simulink model "syncMachVsSwing_sim"  (R2014b)
settings: Solver=ode45  SolverMode=SingleTasking  StartTime=0.0  StopTime=10  MaxStep=0.001  RelTol=0.0001
values from neighbouring files (symbols this model uses):
  cc1 = 2*Ld*Lff - 3*Laf^2    (= 0.0506605918212)    [syncMachVsSwing.m]
  Ert = mpcA.gen([2 3],VG)*baseV    [ex14busSGandPV.m]    (also in ex7busLongLine.m = 24200; exDroopA.m = mpc.bus(ssgen,VM).*baseV(ssgen); exDroopB.m = mpc.bus(ssgen,VM).*baseV(ssgen); exSyncGenPVinv.m = Ert( [1:(synrp-1),(synrp+1):end]  ))
  If_dc = 0.2*Prt./Ert    [ex14busSGandPV.m]    (also in ex7busLongLine.m = Prt./(60*Vf_dc); exDroopA.m = Prt./(60*Vf_dc); exDroopB.m = Prt./(60*Vf_dc); exSyncGenPVinv.m)
  Kd = KD_GAIN_CNST*J*ws    [ex14busSGandPV.m]    (also in ex2busStability.m = 24000; ex7busLongLine.m; ex9busSG.m; exDroopA.m)
  L0 = 0.1*Ld    [ex14busSGandPV.m]    (also in ex7busLongLine.m; exDroopA.m; exDroopB.m; exSyncGenPVinv.m)
  Laf = (2^0.5)*Ert./(ws*If_dc)    [ex14busSGandPV.m]    (also in ex7busLongLine.m; exDroopA.m; exDroopB.m; exSyncGenPVinv.m = (2^0.5)*5*Ert.^2./(ws*Prt))
  Ld = 0.6*Lpu    [ex14busSGandPV.m]    (also in ex7busLongLine.m = 0.3*Lpu; exDroopA.m = 0.3*Lpu; exDroopB.m = 0.3*Lpu; exSyncGenPVinv.m)
  Lff = 2*Laf.^2./Ld    [ex14busSGandPV.m]    (also in ex7busLongLine.m; exDroopA.m; exDroopB.m; exSyncGenPVinv.m)
  Lq = Ld    [ex14busSGandPV.m]    (also in ex7busLongLine.m; exDroopA.m; exDroopB.m; exSyncGenPVinv.m)
  Ls = (Ld+Lq)/2    [ex14busSGandPV.m]    (also in ex7busLongLine.m; ex9busSG.m = 3*(Vn_gens.^2) ./ (ws*Pmax_gens); exDroopA.m; exDroopB.m)
  Pm_rt = 3*Prt    [ex14busSGandPV.m]    (also in ex7busLongLine.m = 450000000; exDroopA.m; exDroopB.m; syncMachVsSwing.m = 30000000)
  poles_2Jws = poles./(2*J*ws)    [ex14busSGandPV.m]    (also in ex2busStability.m = poles./(2*ws*J); ex7busLongLine.m; ex9busSG.m = poles./(2*ws*J); exDroopA.m)
  Ra = 0.05*Ert.^2./Prt    [ex14busSGandPV.m]    (also in ex7busLongLine.m = 0.01*Ert.^2./Prt; exDroopA.m = 0.01*Ert.^2./Prt; exDroopB.m = 0.01*Ert.^2./Prt; exSyncGenPVinv.m)
  rel_step = 0.6    [ex3busPV.m]    (also in exLongLinePV.m = 0.02; syncMachVsSwing.m = 1)
  Rf = Lff/1.2    [ex14busSGandPV.m]    (also in ex7busLongLine.m = Vf_dc./If_dc; exDroopA.m = Vf_dc./If_dc; exDroopB.m = Vf_dc./If_dc; exSyncGenPVinv.m)
  step_time = 9    [ex2busStability.m]    (also in ex3busPV.m = 0.05; exDroopB.m = 10; exLongLinePV.m = 1; syncMachVsSwing.m = 5)
  Vf_dc = If_dc.*Rf    [ex14busSGandPV.m]    (also in ex7busLongLine.m = 500 * ones(size(Ert)); exDroopA.m = 500 * ones(size(Ert)); exDroopB.m = 500 * ones(size(Ert)); exSyncGenPVinv.m)
  ws = 2*pi*50    (= 314.159265359)    [ex14busSGandPV.m]    (also in ex2busStability.m; ex3busPV.m; ex7busLongLine.m; ex9busSG.m)
settings Model: Creator=COPEC  LastModifiedBy=Juri
settings OptimizationCC: BlockReduction=off  BooleanDataType=off
settings DebuggingCC: SaveWithParameterizedLinksMsg=none  UnderspecifiedInitializationDetection=Classic  MergeDetectMultiDrivingBlocksExec=none  SignalResolutionControl=TryResolveAllWithWarning  SolverPrmCheckMsg=none  FrameProcessingCompatibilityMsg=error
settings HardwareCC: TargetUnknown=on

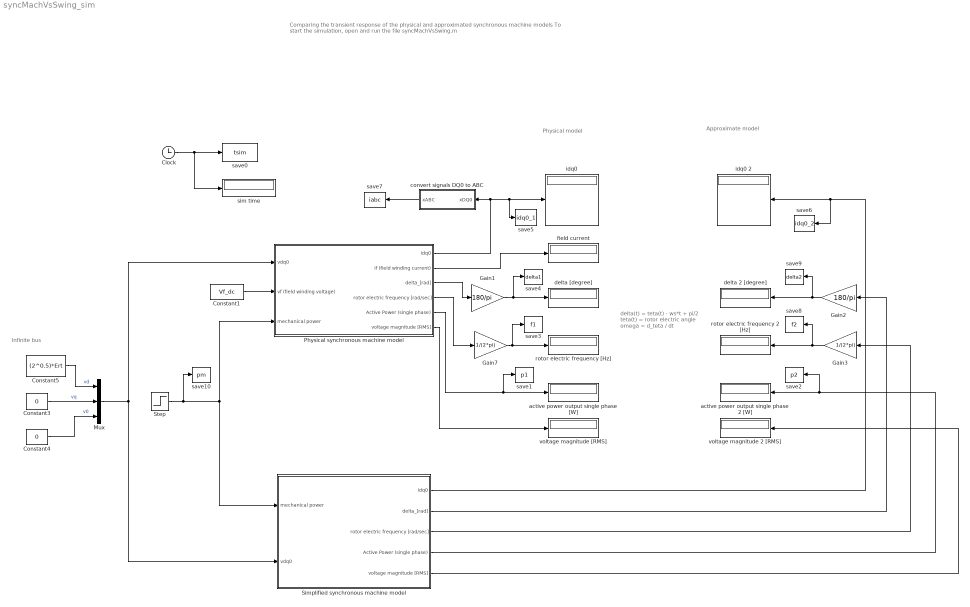
== system syncMachVsSwing_sim ==
  note: Physical
      | model
  note: Comparing the transient response of the physical and approximated synchronous machine models
      |
      | To start the simulation, open and run the file
      | syncMachVsSwing.m
  note: Infinite bus
  note: delta(t) = teta(t) - ws*t + pi/2
      | teta(t) = rotor electric angle
      | omega = d_teta / dt
  note: Approximate model
  Clock : Clock
  Constant1 : Constant  Value=Vf_dc
  Constant3 : Constant  Value=0
  Constant4 : Constant  Value=0
  Constant5 : Constant  Value=(2^0.5)*Ert
  Gain1 : Gain  Gain=180/pi
  Gain2 : Gain  Gain=180/pi
  Gain3 : Gain  Gain=1/(2*pi)
  Gain7 : Gain  Gain=1/(2*pi)
  Mux : Mux  Inputs=3
  Physical synchronous machine model : Subsystem
  Simplified synchronous machine model : Subsystem
  Step : Step  Time=step_time  Before=0.5*Pm_rt  After=0.5*Pm_rt*(1+rel_step)  SampleTime=0
  active power output single phase 2 [W] : Display
  active power output single phase [W] : Display
  "convert signals DQ0 to ABC " : Subsystem
  delta 2 [degree] : Display
  delta [degree] : Display
  field current : Display
  idq0 : Display
  idq0 2 : Display
  rotor electric frequency 2 [Hz] : Display
  rotor electric frequency [Hz] : Display
  save0 : ToWorkspace  VariableName=tsim  SampleTime=-1
  save1 : ToWorkspace  VariableName=p1  SampleTime=-1
  save10 : ToWorkspace  VariableName=pm  SampleTime=-1
  save2 : ToWorkspace  VariableName=p2  SampleTime=-1
  save3 : ToWorkspace  VariableName=f1  SampleTime=-1
  save4 : ToWorkspace  VariableName=delta1  SampleTime=-1
  save5 : ToWorkspace  VariableName=idq0_1  SampleTime=-1
  save6 : ToWorkspace  VariableName=idq0_2  SampleTime=-1
  save7 : ToWorkspace  VariableName=iabc  SampleTime=-1
  save8 : ToWorkspace  VariableName=f2  SampleTime=-1
  save9 : ToWorkspace  VariableName=delta2  SampleTime=-1
  sim time : Display
  voltage magnitude 2 [RMS] : Display
  voltage magnitude [RMS] : Display
  wires:
  Clock/1 -> sim time/1, save0/1
  Constant1/1 -> Physical synchronous machine model/2(vf (field winding voltage))
  Step/1 -> save10/1, Physical synchronous machine model/3(mechanical power), Simplified synchronous machine model/1(mechanical power)
  Physical synchronous machine model/1(idq0) -> "convert signals DQ0 to ABC "/1(xDQ0), save5/1, idq0/1
  Physical synchronous machine model/2(if (field winding current)) -> field current/1
  Physical synchronous machine model/3(delta_[rad]) -> Gain1/1
  Physical synchronous machine model/4(rotor electric frequency [rad/sec]) -> Gain7/1
  Gain1/1 -> save4/1, delta [degree]/1
  Gain7/1 -> save3/1, rotor electric frequency [Hz]/1
  Physical synchronous machine model/5(Active Power (single phase)) -> save1/1, active power output single phase [W]/1
  Physical synchronous machine model/6(voltage magnitude [RMS]) -> voltage magnitude [RMS]/1
  Constant5/1 -> Mux/1  "vd"
  Constant3/1 -> Mux/2  "vq"
  Constant4/1 -> Mux/3  "v0"
  Mux/1 -> Simplified synchronous machine model/2(vdq0), Physical synchronous machine model/1(vdq0)
  "convert signals DQ0 to ABC "/1(xABC) -> save7/1
  Gain2/1 -> save9/1, delta 2 [degree]/1
  Gain3/1 -> save8/1, rotor electric frequency 2 [Hz]/1
  Simplified synchronous machine model/1(idq0) -> save6/1, idq0 2/1
  Simplified synchronous machine model/2(delta_[rad]) -> Gain2/1
  Simplified synchronous machine model/3(rotor electric frequency [rad/sec]) -> Gain3/1
  Simplified synchronous machine model/4(Active Power (single phase)) -> save2/1, active power output single phase 2 [W]/1
  Simplified synchronous machine model/5(voltage magnitude [RMS]) -> voltage magnitude 2 [RMS]/1

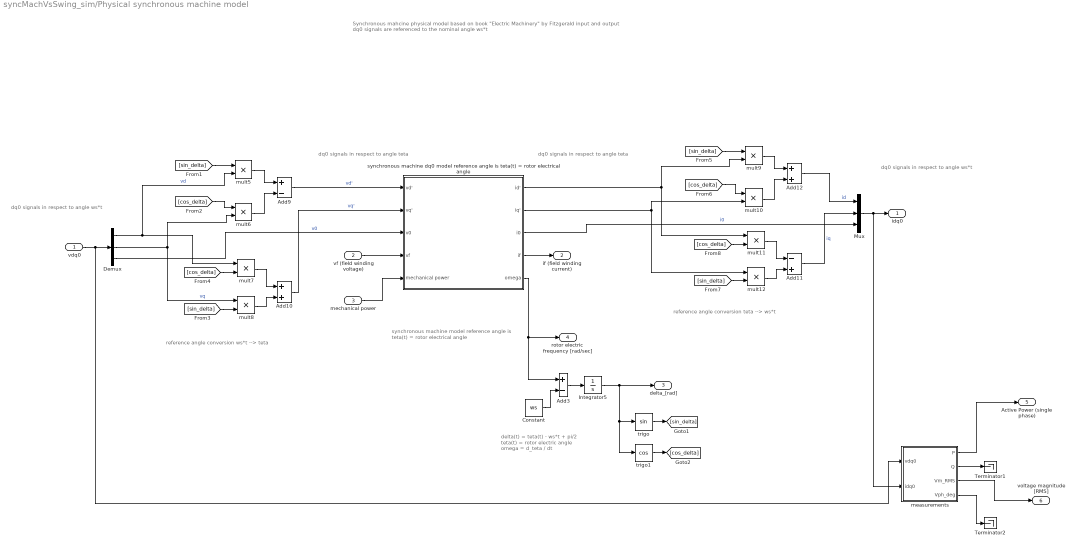
== system syncMachVsSwing_sim/Physical synchronous machine model ==
  note: Synchronous mahcine physical model
      | based on book "Electric Machinery" by Fitzgerald
      |
      | input and output dq0 signals are referenced
      | to the nominal angle ws*t
  note: reference angle conversion ws*t --> teta
  note: synchronous machine model
      | reference angle is
      | teta(t) = rotor electrical angle
  note: reference angle conversion teta --> ws*t
  note: dq0 signals in respect to angle ws*t
  note: dq0 signals in respect to angle ws*t
  note: dq0 signals in respect to angle teta
  note: dq0 signals in respect to angle teta
  note: delta(t) = teta(t) - ws*t + pi/2
      | teta(t) = rotor electric angle
      | omega = d_teta / dt
  vdq0 : Inport
  vf (field winding voltage) : Inport  Port=2
  mechanical power : Inport  Port=3
  Add10 : Sum
  Add11 : Sum  Inputs=-+
  Add12 : Sum
  Add3 : Sum  Inputs=+-
  Add9 : Sum  Inputs=+-
  Constant : Constant  Value=ws
  Demux : Demux  Outputs=3
  Integrator5 : Integrator
  Mux : Mux  Inputs=3
  Terminator1 : Terminator
  Terminator2 : Terminator
  measurements : Subsystem
  mult{5..12} (8 alike) : Product  Inputs=**
  synchronous machine dq0 model reference angle is teta(t) = rotor electrical angle : Subsystem
  trigo : Trigonometry
  trigo1 : Trigonometry  Operator=cos
  idq0 : Outport
  if (field winding current) : Outport  Port=2
  delta_[rad] : Outport  Port=3
  rotor electric frequency [rad/sec] : Outport  Port=4
  Active Power (single phase) : Outport  Port=5
  voltage magnitude [RMS] : Outport  Port=6
  wires:
  vdq0/1 -> measurements/1(vdq0), Demux/1
  Demux/1 -> mult5/2, mult7/1  "vd"
  Demux/2 -> mult6/2, mult8/1  "vq"
  mult5/1 -> Add9/1
  mult6/1 -> Add9/2
  [sin_delta] -> mult5/1
  [cos_delta] -> mult6/1
  mult7/1 -> Add10/1
  mult8/1 -> Add10/2
  [cos_delta] -> mult7/2
  [sin_delta] -> mult8/2
  mult9/1 -> Add12/1
  mult10/1 -> Add12/2
  [sin_delta] -> mult9/1
  [cos_delta] -> mult10/1
  mult11/1 -> Add11/1
  mult12/1 -> Add11/2
  [cos_delta] -> mult11/2
  [sin_delta] -> mult12/2
  Mux/1 -> measurements/2(idq0), idq0/1
  Add11/1 -> Mux/2  "iq"
  Add12/1 -> Mux/1  "id"
  synchronous machine dq0 model reference angle is teta(t) = rotor electrical angle/1(id') -> mult11/1, mult9/2
  synchronous machine dq0 model reference angle is teta(t) = rotor electrical angle/2(iq') -> mult12/1, mult10/2
  Add9/1 -> synchronous machine dq0 model reference angle is teta(t) = rotor electrical angle/1(vd')  "vd'"
  mechanical power/1 -> synchronous machine dq0 model reference angle is teta(t) = rotor electrical angle/5(mechanical power)
  Demux/3 -> synchronous machine dq0 model reference angle is teta(t) = rotor electrical angle/3(v0)  "v0"
  Add10/1 -> synchronous machine dq0 model reference angle is teta(t) = rotor electrical angle/2(vq')  "vq'"
  vf (field winding voltage)/1 -> synchronous machine dq0 model reference angle is teta(t) = rotor electrical angle/4(vf)
  synchronous machine dq0 model reference angle is teta(t) = rotor electrical angle/3(i0) -> Mux/3  "i0"
  synchronous machine dq0 model reference angle is teta(t) = rotor electrical angle/4(if) -> if (field winding current)/1
  trigo/1 -> [sin_delta]
  trigo1/1 -> [cos_delta]
  Add3/1 -> Integrator5/1
  Constant/1 -> Add3/2
  synchronous machine dq0 model reference angle is teta(t) = rotor electrical angle/5(omega) -> Add3/1, rotor electric frequency [rad/sec]/1
  Integrator5/1 -> delta_[rad]/1, trigo1/1, trigo/1
  measurements/1(P) -> Active Power (single phase)/1
  measurements/2(Q) -> Terminator1/1
  measurements/3(Vm_RMS) -> voltage magnitude [RMS]/1
  measurements/4(Vph_deg) -> Terminator2/1

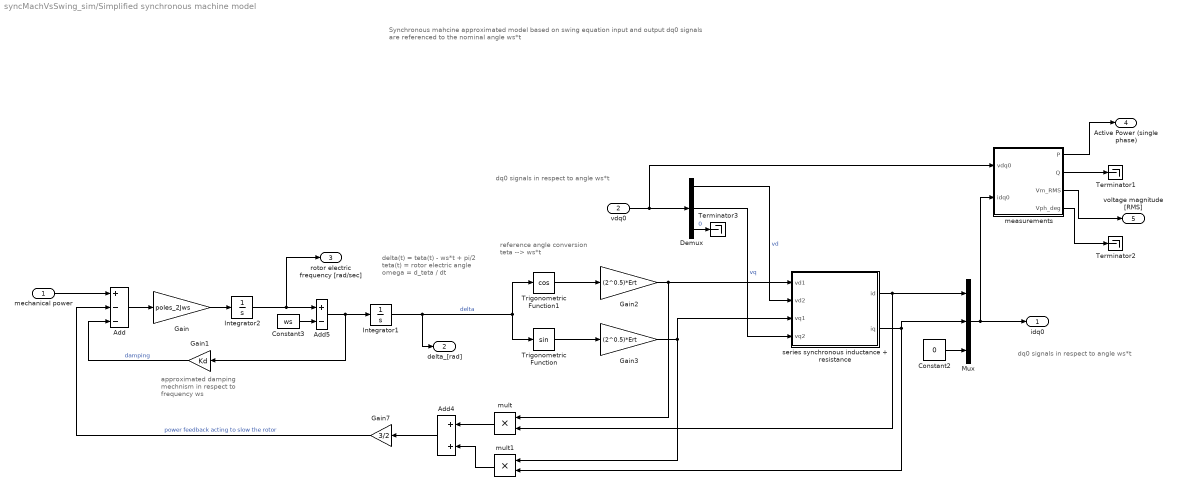
== system syncMachVsSwing_sim/Simplified synchronous machine model ==
  note: reference angle conversion
      | teta --> ws*t
  note: approximated damping
      | mechnism in respect to
      | frequency ws
  note: delta(t) = teta(t) - ws*t + pi/2
      | teta(t) = rotor electric angle
      | omega = d_teta / dt
  note: dq0 signals in respect to angle ws*t
  note: dq0 signals in respect to angle ws*t
  note: Synchronous mahcine approximated model
      | based on swing equation
      |
      | input and output dq0 signals are referenced
      | to the nominal angle ws*t
  mechanical power : Inport
  vdq0 : Inport  Port=2
  Add : Sum  Inputs=+--
  Add4 : Sum
  Add5 : Sum  Inputs=+-
  Constant2 : Constant  Value=0
  Constant3 : Constant  Value=ws
  Demux : Demux  Outputs=3
  Gain : Gain  Gain=poles_2Jws
  Gain1 : Gain  Gain=Kd
  Gain2 : Gain  Gain=(2^0.5)*Ert
  Gain3 : Gain  Gain=(2^0.5)*Ert
  Gain7 : Gain  Gain=3/2
  Integrator1 : Integrator
  Integrator2 : Integrator  InitialCondition=ws
  Mux : Mux  Inputs=3
  Terminator1 : Terminator
  Terminator2 : Terminator
  Terminator3 : Terminator
  Trigonometric Function : Trigonometry
  Trigonometric Function1 : Trigonometry  Operator=cos
  measurements : Subsystem
  mult : Product  Inputs=**
  mult1 : Product  Inputs=**
  series synchronous inductance + resistance : Subsystem
  idq0 : Outport
  delta_[rad] : Outport  Port=2
  rotor electric frequency [rad/sec] : Outport  Port=3
  Active Power (single phase) : Outport  Port=4
  voltage magnitude [RMS] : Outport  Port=5
  wires:
  mechanical power/1 -> Add/1
  Add/1 -> Gain/1
  Gain/1 -> Integrator2/1
  Integrator1/1 -> delta_[rad]/1, Trigonometric Function1/1, Trigonometric Function/1  "delta"
  Gain1/1 -> Add/3  "damping"
  mult/1 -> Add4/1
  mult1/1 -> Add4/2
  Add4/1 -> Gain7/1
  Gain7/1 -> Add/2  "power feedback acting to slow the rotor"
  Constant2/1 -> Mux/3
  measurements/1(P) -> Active Power (single phase)/1
  measurements/2(Q) -> Terminator1/1
  measurements/3(Vm_RMS) -> voltage magnitude [RMS]/1
  measurements/4(Vph_deg) -> Terminator2/1
  Gain2/1 -> mult/1, series synchronous inductance + resistance/1(vd1)
  Gain3/1 -> mult1/1, series synchronous inductance + resistance/3(vq1)
  vdq0/1 -> Demux/1, measurements/1(vdq0)
  Demux/1 -> series synchronous inductance + resistance/2(vd2)  "vd"
  Demux/2 -> series synchronous inductance + resistance/4(vq2)  "vq"
  Demux/3 -> Terminator3/1  "0"
  Mux/1 -> measurements/2(idq0), idq0/1
  series synchronous inductance + resistance/1(id) -> mult/2, Mux/1
  series synchronous inductance + resistance/2(iq) -> mult1/2, Mux/2
  Integrator2/1 -> Add5/1, rotor electric frequency [rad/sec]/1
  Add5/1 -> Gain1/1, Integrator1/1
  Constant3/1 -> Add5/2
  Trigonometric Function1/1 -> Gain2/1
  Trigonometric Function/1 -> Gain3/1

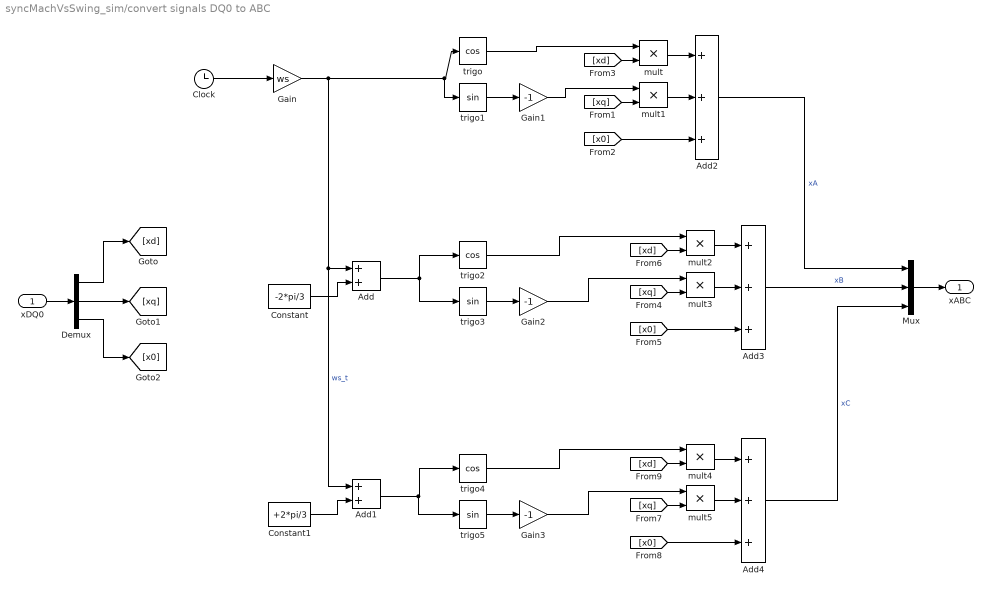
== system syncMachVsSwing_sim/convert signals DQ0 to ABC  ==
  xDQ0 : Inport
  Add : Sum
  Add1 : Sum
  Add2 : Sum  Inputs=+++
  Add3 : Sum  Inputs=+++
  Add4 : Sum  Inputs=+++
  Clock : Clock
  Constant : Constant  Value=-2*pi/3
  Constant1 : Constant  Value=+2*pi/3
  Demux : Demux  Outputs=3
  Gain : Gain  Gain=ws
  Gain1 : Gain  Gain=-1
  Gain2 : Gain  Gain=-1
  Gain3 : Gain  Gain=-1
  Mux : Mux  Inputs=3
  mult{,1..5} (6 alike) : Product  Inputs=**
  trigo : Trigonometry  Operator=cos
  trigo1 : Trigonometry
  trigo2 : Trigonometry  Operator=cos
  trigo3 : Trigonometry
  trigo4 : Trigonometry  Operator=cos
  trigo5 : Trigonometry
  xABC : Outport
  wires:
  Clock/1 -> Gain/1
  Gain/1 -> trigo1/1, trigo/1, Add1/1, Add/1  "ws_t"
  Constant/1 -> Add/2
  Constant1/1 -> Add1/2
  trigo1/1 -> Gain1/1
  trigo3/1 -> Gain2/1
  Add/1 -> trigo2/1, trigo3/1
  trigo5/1 -> Gain3/1
  Add1/1 -> trigo5/1, trigo4/1
  xDQ0/1 -> Demux/1
  Demux/1 -> [xd]
  Demux/2 -> [xq]
  Demux/3 -> [x0]
  Mux/1 -> xABC/1
  mult/1 -> Add2/1
  mult1/1 -> Add2/2
  [xd] -> mult/2
  [xq] -> mult1/2
  [x0] -> Add2/3
  mult2/1 -> Add3/1
  mult3/1 -> Add3/2
  [xd] -> mult2/2
  [xq] -> mult3/2
  [x0] -> Add3/3
  mult4/1 -> Add4/1
  mult5/1 -> Add4/2
  [xd] -> mult4/2
  [xq] -> mult5/2
  [x0] -> Add4/3
  trigo/1 -> mult/1
  Gain1/1 -> mult1/1
  trigo2/1 -> mult2/1
  Gain2/1 -> mult3/1
  trigo4/1 -> mult4/1
  Gain3/1 -> mult5/1
  Add2/1 -> Mux/1  "xA"
  Add3/1 -> Mux/2  "xB"
  Add4/1 -> Mux/3  "xC"

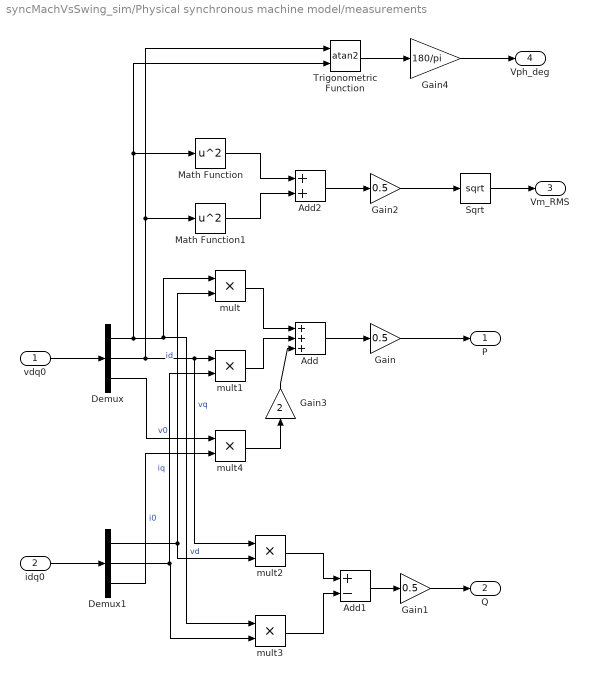
== system syncMachVsSwing_sim/Physical synchronous machine model/measurements ==
  vdq0 : Inport
  idq0 : Inport  Port=2
  Add : Sum  Inputs=+++
  Add1 : Sum  Inputs=+-
  Add2 : Sum
  Demux : Demux  Outputs=3
  Demux1 : Demux  Outputs=3
  Gain : Gain  Gain=0.5
  Gain1 : Gain  Gain=0.5
  Gain2 : Gain  Gain=0.5
  Gain3 : Gain  Gain=2
  Gain4 : Gain  Gain=180/pi
  Math Function : Math  Operator=square  SaturateOnIntegerOverflow=on
  Math Function1 : Math  Operator=square  SaturateOnIntegerOverflow=on
  Sqrt : Sqrt  SaturateOnIntegerOverflow=on
  Trigonometric Function : Trigonometry  Operator=atan2
  mult{,1..4} (5 alike) : Product  Inputs=**
  P : Outport
  Q : Outport  Port=2
  Vm_RMS : Outport  Port=3
  Vph_deg : Outport  Port=4
  wires:
  idq0/1 -> Demux1/1
  vdq0/1 -> Demux/1
  Demux/1 -> Math Function/1, Trigonometric Function/2, mult3/1, mult/1  "vd"
  Demux/2 -> Trigonometric Function/1, Math Function1/1, mult2/1, mult1/1  "vq"
  Demux1/1 -> mult/2, mult2/2  "id"
  Demux1/2 -> mult3/2, mult1/2  "iq"
  Demux/3 -> mult4/1  "v0"
  Demux1/3 -> mult4/2  "i0"
  mult/1 -> Add/1
  mult1/1 -> Add/2
  Add/1 -> Gain/1
  mult2/1 -> Add1/1
  mult3/1 -> Add1/2
  Add1/1 -> Gain1/1
  Sqrt/1 -> Vm_RMS/1
  Math Function/1 -> Add2/1
  Math Function1/1 -> Add2/2
  Add2/1 -> Gain2/1
  Gain2/1 -> Sqrt/1
  Gain/1 -> P/1
  Gain1/1 -> Q/1
  mult4/1 -> Gain3/1
  Gain3/1 -> Add/3
  Trigonometric Function/1 -> Gain4/1
  Gain4/1 -> Vph_deg/1

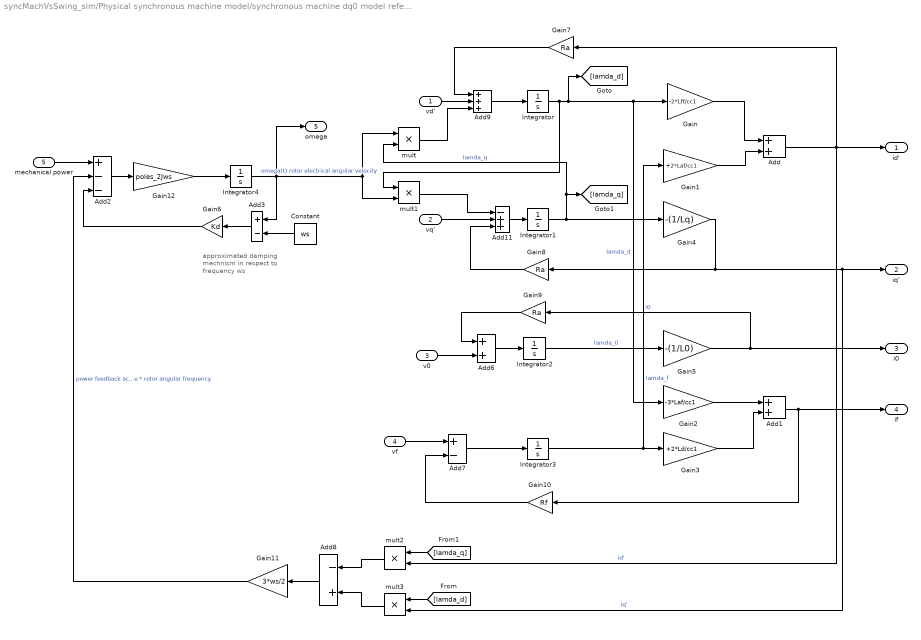
== system syncMachVsSwing_sim/Physical synchronous machine model/synchronous machine dq0 model reference angle is teta(t) = rotor electrical angle ==
  note: approximated damping
      | mechnism in respect to
      | frequency ws
  vd' : Inport
  vq' : Inport  Port=2
  v0 : Inport  Port=3
  vf : Inport  Port=4
  mechanical power : Inport  Port=5
  Add : Sum
  Add1 : Sum
  Add11 : Sum  Inputs=-++
  Add2 : Sum  Inputs=+--
  Add3 : Sum  Inputs=+-
  Add6 : Sum
  Add7 : Sum  Inputs=+-
  Add8 : Sum  Inputs=-+
  Add9 : Sum  Inputs=+++
  Constant : Constant  Value=ws
  Gain : Gain  Gain=-2*Lff/cc1
  Gain1 : Gain  Gain=+2*Laf/cc1
  Gain10 : Gain  Gain=Rf
  Gain11 : Gain  Gain=3*ws/2
  Gain12 : Gain  Gain=poles_2Jws
  Gain2 : Gain  Gain=-3*Laf/cc1
  Gain3 : Gain  Gain=+2*Ld/cc1
  Gain4 : Gain  Gain=-(1/Lq)
  Gain5 : Gain  Gain=-(1/L0)
  Gain6 : Gain  Gain=Kd
  Gain7 : Gain  Gain=Ra
  Gain8 : Gain  Gain=Ra
  Gain9 : Gain  Gain=Ra
  Integrator : Integrator
  Integrator1 : Integrator
  Integrator2 : Integrator
  Integrator3 : Integrator  InitialCondition=Lff*If_dc
  Integrator4 : Integrator  InitialCondition=ws
  mult{,1..3} (4 alike) : Product  Inputs=**
  id' : Outport
  iq' : Outport  Port=2
  i0 : Outport  Port=3
  if : Outport  Port=4
  omega : Outport  Port=5
  wires:
  Gain1/1 -> Add/2
  Add6/1 -> Integrator2/1
  mechanical power/1 -> Add2/1
  Gain6/1 -> Add2/3
  Integrator/1 -> mult1/1, Gain2/1, Gain/1, [lamda_d]  "lamda_d"
  Gain5/1 -> i0/1, Gain9/1  "i0"
  Integrator1/1 -> Gain4/1, [lamda_q], mult/2  "lamda_q"
  Integrator2/1 -> Gain5/1  "lamda_0"
  Integrator3/1 -> Gain1/1, Gain3/1  "lamda_f"
  Add1/1 -> if/1, Gain10/1
  Gain4/1 -> iq'/1, mult3/2, Gain8/1  "iq'"
  Add/1 -> mult2/2, id'/1, Gain7/1  "id'"
  Gain/1 -> Add/1
  vf/1 -> Add7/1
  Add7/1 -> Integrator3/1
  Gain9/1 -> Add6/1
  Add8/1 -> Gain11/1
  Gain11/1 -> Add2/2  "power feedback acting to slow the rotor = Torque * rotor angular frequency"
  Gain8/1 -> Add11/3
  mult/1 -> Add9/3
  mult1/1 -> Add11/1
  Add9/1 -> Integrator/1
  vd'/1 -> Add9/2
  Gain3/1 -> Add1/2
  Gain2/1 -> Add1/1
  Gain10/1 -> Add7/2
  Add11/1 -> Integrator1/1
  Gain7/1 -> Add9/1
  mult3/1 -> Add8/2
  mult2/1 -> Add8/1
  v0/1 -> Add6/2
  Add3/1 -> Gain6/1
  Constant/1 -> Add3/2
  vq'/1 -> Add11/2
  [lamda_q] -> mult2/1
  [lamda_d] -> mult3/1
  Integrator4/1 -> omega/1, Add3/1, mult1/2, mult/1  "omega(t) rotor electrical angular velocity"
  Add2/1 -> Gain12/1
  Gain12/1 -> Integrator4/1

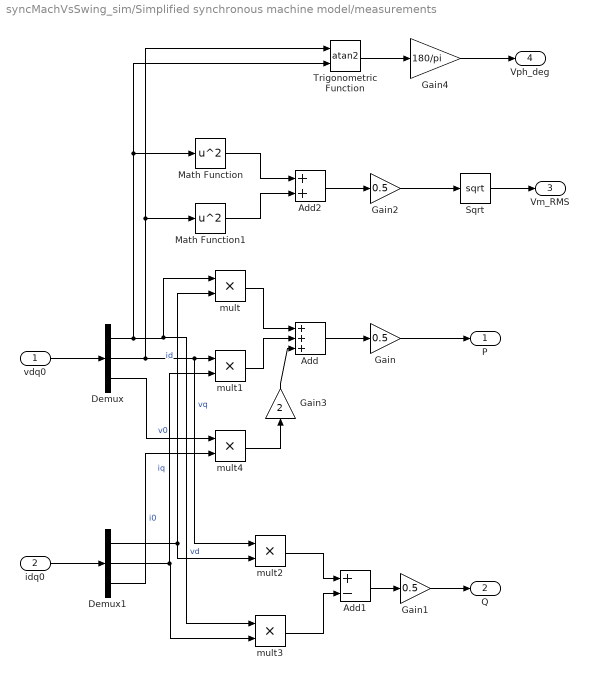
== system syncMachVsSwing_sim/Simplified synchronous machine model/measurements ==
  vdq0 : Inport
  idq0 : Inport  Port=2
  Add : Sum  Inputs=+++
  Add1 : Sum  Inputs=+-
  Add2 : Sum
  Demux : Demux  Outputs=3
  Demux1 : Demux  Outputs=3
  Gain : Gain  Gain=0.5
  Gain1 : Gain  Gain=0.5
  Gain2 : Gain  Gain=0.5
  Gain3 : Gain  Gain=2
  Gain4 : Gain  Gain=180/pi
  Math Function : Math  Operator=square  SaturateOnIntegerOverflow=on
  Math Function1 : Math  Operator=square  SaturateOnIntegerOverflow=on
  Sqrt : Sqrt  SaturateOnIntegerOverflow=on
  Trigonometric Function : Trigonometry  Operator=atan2
  mult{,1..4} (5 alike) : Product  Inputs=**
  P : Outport
  Q : Outport  Port=2
  Vm_RMS : Outport  Port=3
  Vph_deg : Outport  Port=4
  wires:
  idq0/1 -> Demux1/1
  vdq0/1 -> Demux/1
  Demux/1 -> Math Function/1, Trigonometric Function/2, mult3/1, mult/1  "vd"
  Demux/2 -> Trigonometric Function/1, Math Function1/1, mult2/1, mult1/1  "vq"
  Demux1/1 -> mult/2, mult2/2  "id"
  Demux1/2 -> mult3/2, mult1/2  "iq"
  Demux/3 -> mult4/1  "v0"
  Demux1/3 -> mult4/2  "i0"
  mult/1 -> Add/1
  mult1/1 -> Add/2
  Add/1 -> Gain/1
  mult2/1 -> Add1/1
  mult3/1 -> Add1/2
  Add1/1 -> Gain1/1
  Sqrt/1 -> Vm_RMS/1
  Math Function/1 -> Add2/1
  Math Function1/1 -> Add2/2
  Add2/1 -> Gain2/1
  Gain2/1 -> Sqrt/1
  Gain/1 -> P/1
  Gain1/1 -> Q/1
  mult4/1 -> Gain3/1
  Gain3/1 -> Add/3
  Trigonometric Function/1 -> Gain4/1
  Gain4/1 -> Vph_deg/1

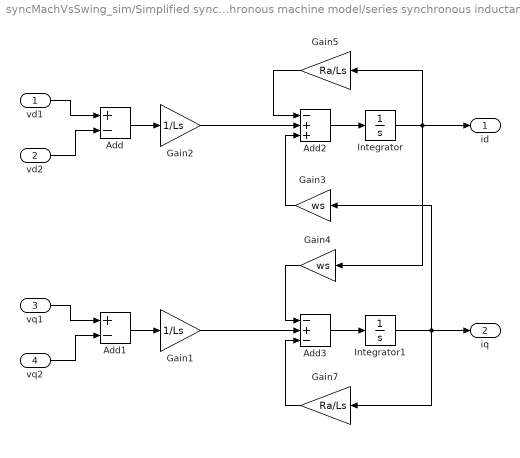
== system syncMachVsSwing_sim/Simplified synchronous machine model/series synchronous inductance + resistance ==
  vd1 : Inport
  vd2 : Inport  Port=2
  vq1 : Inport  Port=3
  vq2 : Inport  Port=4
  Add : Sum  Inputs=+-
  Add1 : Sum  Inputs=+-
  Add2 : Sum  Inputs=-++
  Add3 : Sum  Inputs=-+-
  Gain1 : Gain  Gain=1/Ls
  Gain2 : Gain  Gain=1/Ls
  Gain3 : Gain  Gain=ws
  Gain4 : Gain  Gain=ws
  Gain5 : Gain  Gain=Ra/Ls
  Gain7 : Gain  Gain=Ra/Ls
  Integrator : Integrator
  Integrator1 : Integrator
  id : Outport
  iq : Outport  Port=2
  wires:
  vd1/1 -> Add/1
  vd2/1 -> Add/2
  vq1/1 -> Add1/1
  vq2/1 -> Add1/2
  Add/1 -> Gain2/1
  Add1/1 -> Gain1/1
  Integrator/1 -> Gain4/1, id/1, Gain5/1
  Integrator1/1 -> Gain7/1, Gain3/1, iq/1
  Add2/1 -> Integrator/1
  Add3/1 -> Integrator1/1
  Gain3/1 -> Add2/3
  Gain2/1 -> Add2/2
  Gain4/1 -> Add3/1
  Gain1/1 -> Add3/2
  Gain5/1 -> Add2/1
  Gain7/1 -> Add3/3
